simulink model "Milestone3"  (R2022a)
settings: Solver=FixedStepAuto  StartTime=0.0  StopTime=5000  RelTol=1e-3
undefined symbols (not defined in the file or in its folder): InputPWM, WheelSpeed
libraries: arduinolib x20, mobileRoboticsTrainingLib x2
settings Model: ExtModeTrigDuration=2  Creator=sarah  LastModifiedBy=sarah
settings OptimizationCC: EnhancedBackFolding=on  PassReuseOutputArgsAs=Individual arguments  ZeroExternalMemoryAtStartup=off  ZeroInternalMemoryAtStartup=off  MaxStackSize=64  OptimizeBlockOrder=speed  DifferentSizesBufferReuse=on  OptimizationCustomize=off  EfficientTunableParamExpr=on
settings DebuggingCC: ParameterTunabilityLossMsg=error
settings HardwareCC: ProdBitPerPointer=32  ProdBitPerSizeT=32  ProdBitPerPtrDiffT=32  ProdLargestAtomicInteger=Long  ProdLargestAtomicFloat=Double  ProdWordSize=32  ProdHWDeviceType=ARM Compatible->ARM Cortex  UseEmbeddedCoderFeatures=off  UseSimulinkCoderFeatures=off
settings SFSimCC: MATLABDynamicMemAlloc=off
settings RTWCC: SystemTargetFile=ert.tlc  HardwareBoard=Arduino Nano 33 IoT  TemplateMakefile=ert_default_tmf  Toolchain=Arduino ARM
settings CodeAppCC: ForceParamTrailComments=on  IgnoreCustomStorageClasses=off  OperatorAnnotations=on  SimulinkDataObjDesc=on  SFDataObjDesc=on  InsertBlockDesc=on
settings ERTTargetCC: SupportContinuousTime=on  SupportNonInlinedSFcns=on  SupportVariableSizeSignals=on  ExtModeTransport=3  ExtModeStaticAlloc=on  ExtModeStaticAllocSize=8192  ExtModeMexFile=ext_xcp  ExtModeIntrfLevel=Level2 - Open

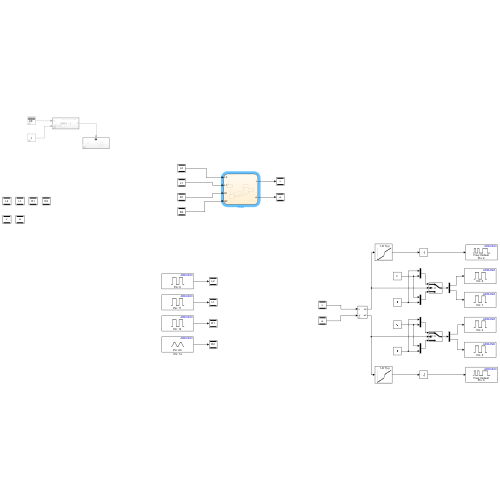
[thumbnail: Simulink's stored preview of the top-level diagram]
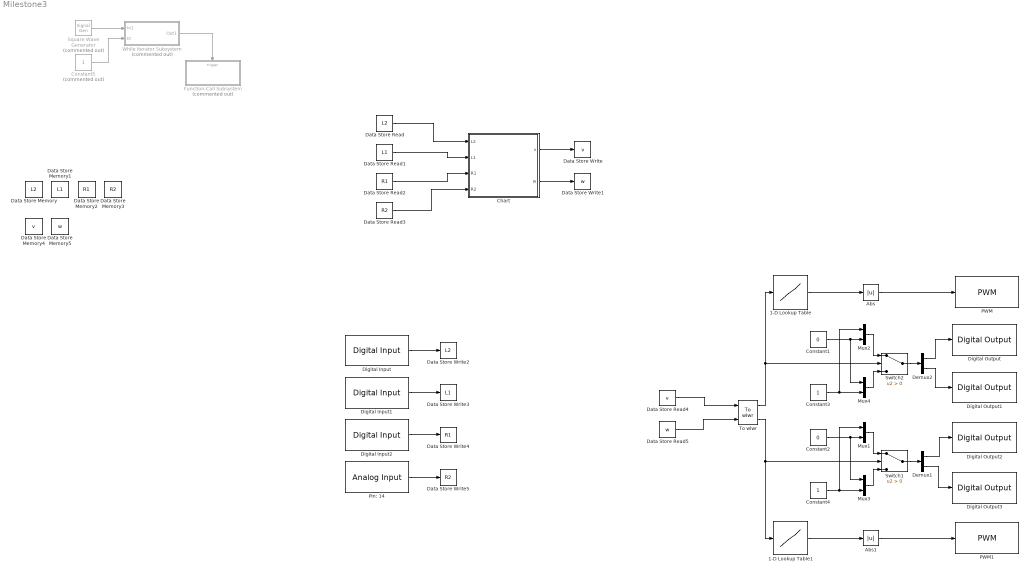
== system Milestone3 ==
  1-D Lookup Table : Lookup_n-D  NumberOfTableDimensions=1  BreakpointsForDimension1=WheelSpeed  Table=InputPWM  InternalRulePriority=Speed  RndMeth=Simplest
  1-D Lookup Table1 : Lookup_n-D  NumberOfTableDimensions=1  BreakpointsForDimension1=WheelSpeed  Table=InputPWM  InternalRulePriority=Speed  RndMeth=Simplest
  Abs : Abs  SaturateOnIntegerOverflow=off
  Abs1 : Abs  SaturateOnIntegerOverflow=off
  Chart : Stateflow chart  TreatAsAtomicUnit=on
  Constant1 : Constant  Value=0
  Constant2 : Constant  Value=0
  Constant3 : Constant
  Constant4 : Constant
  Constant5 : Constant  Commented=on
  Data Store Memory : DataStoreMemory  DataStoreName=L2  WriteAfterWriteMsg=warning  ShowAdditionalParam=off
  Data Store Memory1 : DataStoreMemory  DataStoreName=L1  WriteAfterWriteMsg=warning  ShowAdditionalParam=off
  Data Store Memory2 : DataStoreMemory  DataStoreName=R1  WriteAfterWriteMsg=warning  ShowAdditionalParam=off
  Data Store Memory3 : DataStoreMemory  DataStoreName=R2  WriteAfterWriteMsg=warning  ShowAdditionalParam=off
  Data Store Memory4 : DataStoreMemory  DataStoreName=v  WriteAfterWriteMsg=warning  ShowAdditionalParam=off
  Data Store Memory5 : DataStoreMemory  DataStoreName=w  WriteAfterWriteMsg=warning  ShowAdditionalParam=off
  Data Store Read : DataStoreRead  DataStoreName=L2  IndexOptions=Index vector (dialog)  Indices=1  OutputSizes=1
  Data Store Read1 : DataStoreRead  DataStoreName=L1  IndexOptions=Index vector (dialog)  Indices=1  OutputSizes=1
  Data Store Read2 : DataStoreRead  DataStoreName=R1  IndexOptions=Index vector (dialog)  Indices=1  OutputSizes=1
  Data Store Read3 : DataStoreRead  DataStoreName=R2  IndexOptions=Index vector (dialog)  Indices=1  OutputSizes=1
  Data Store Read4 : DataStoreRead  DataStoreName=v  IndexOptions=Index vector (dialog)  Indices=1  OutputSizes=1
  Data Store Read5 : DataStoreRead  DataStoreName=w  IndexOptions=Index vector (dialog)  Indices=1  OutputSizes=1
  Data Store Write : DataStoreWrite  DataStoreName=v  IndexOptions=Index vector (dialog)  Indices=1  OutputSizes=1
  Data Store Write1 : DataStoreWrite  DataStoreName=w  IndexOptions=Index vector (dialog)  Indices=1  OutputSizes=1
  Data Store Write2 : DataStoreWrite  DataStoreName=L2  IndexOptions=Index vector (dialog)  Indices=1  OutputSizes=1
  Data Store Write3 : DataStoreWrite  DataStoreName=L1  IndexOptions=Index vector (dialog)  Indices=1  OutputSizes=1
  Data Store Write4 : DataStoreWrite  DataStoreName=R1  IndexOptions=Index vector (dialog)  Indices=1  OutputSizes=1
  Data Store Write5 : DataStoreWrite  DataStoreName=R2  IndexOptions=Index vector (dialog)  Indices=1  OutputSizes=1
  Demux1 : Demux  Outputs=2
  Demux2 : Demux  Outputs=2
  Digital Input : arduinolib/Digital Input  pinNumber=8  mode=Default  Direction=input  SampleTime=-1  blockPlatform=arduino
  Digital Input1 : arduinolib/Digital Input  pinNumber=11  mode=Default  Direction=input  SampleTime=-1  blockPlatform=arduino
  Digital Input2 : arduinolib/Digital Input  pinNumber=12  mode=Default  Direction=input  SampleTime=-1  blockPlatform=arduino
  Digital Output : arduinolib/Digital Output  pinNumber=6  Direction=output  blockPlatform=arduino
  Digital Output1 : arduinolib/Digital Output  pinNumber=7  Direction=output  blockPlatform=arduino
  Digital Output2 : arduinolib/Digital Output  pinNumber=4  Direction=output  blockPlatform=arduino
  Digital Output3 : arduinolib/Digital Output  pinNumber=5  Direction=output  blockPlatform=arduino
  Function-Call Subsystem : Subsystem  Commented=on  TreatAsAtomicUnit=on
  Mux{1..4} (4 alike) : Mux  Inputs=2
  PWM : arduinolib/PWM  pinNumber=2  frequencyType=Default  desiredFrequency=490.2  achievableFrequency=490.2
  PWM1 : arduinolib/PWM  pinNumber=3  frequencyType=Default  desiredFrequency=490.2  achievableFrequency=490.2
  Pin: 14 : arduinolib/Analog Input  pinNumber=0  ReadResultsOnly=off  ConversionTriggerSource=Software  ExternalTriggerType=uint32( 0 )  OutputDataType=uint16  EnableConversionCompleteNotify=off  EnableOuputStatus=off  SampleTime=-1  blockPlatform=arduino
  Square Wave Generator : SignalGenerator  Commented=on  WaveForm=square  Units=rad/sec
  Switch1 : Switch  Criteria=u2 > Threshold  SaturateOnIntegerOverflow=off  InputSameDT=off
  Switch2 : Switch  Criteria=u2 > Threshold  SaturateOnIntegerOverflow=off  InputSameDT=off
  To wlwr : mobileRoboticsTrainingLib/To wlwr  axleLength=axleLength  wheelR=wheelR
  While Iterator Subsystem : Subsystem  Commented=on  TreatAsAtomicUnit=on
  wires:
  Square Wave Generator/1 -> While Iterator Subsystem/1(In1)
  Constant5/1 -> While Iterator Subsystem/2(IC)
  While Iterator Subsystem/1(Out1) -> Function-Call Subsystem/Trigger
  Chart/1(v) -> Data Store Write/1
  Chart/2(w) -> Data Store Write1/1
  Data Store Read/1 -> Chart/1(L2)
  Data Store Read1/1 -> Chart/2(L1)
  Data Store Read3/1 -> Chart/4(R2)
  Data Store Read2/1 -> Chart/3(R1)
  Pin: 14/1 -> Data Store Write5/1
  To wlwr/1 -> 1-D Lookup Table/1, Switch2/2
  Switch2/1 -> Demux2/1
  Constant1/1 -> Mux4/1, Mux2/2
  Abs1/1 -> PWM1/1
  Constant2/1 -> Mux3/1, Mux1/2
  Mux1/1 -> Switch1/1
  1-D Lookup Table1/1 -> Abs1/1
  Constant3/1 -> Mux2/1, Mux4/2
  Demux2/1 -> Digital Output/1
  Switch1/1 -> Demux1/1
  Abs/1 -> PWM/1
  Constant4/1 -> Mux1/1, Mux3/2
  Demux1/1 -> Digital Output2/1
  Demux1/2 -> Digital Output3/1
  To wlwr/2 -> Switch1/2, 1-D Lookup Table1/1
  Mux3/1 -> Switch1/3
  Mux4/1 -> Switch2/3
  Digital Input1/1 -> Data Store Write3/1
  Digital Input/1 -> Data Store Write2/1
  Mux2/1 -> Switch2/1
  Digital Input2/1 -> Data Store Write4/1
  Demux2/2 -> Digital Output1/1
  Data Store Read4/1 -> To wlwr/1
  1-D Lookup Table/1 -> Abs/1
  Data Store Read5/1 -> To wlwr/2

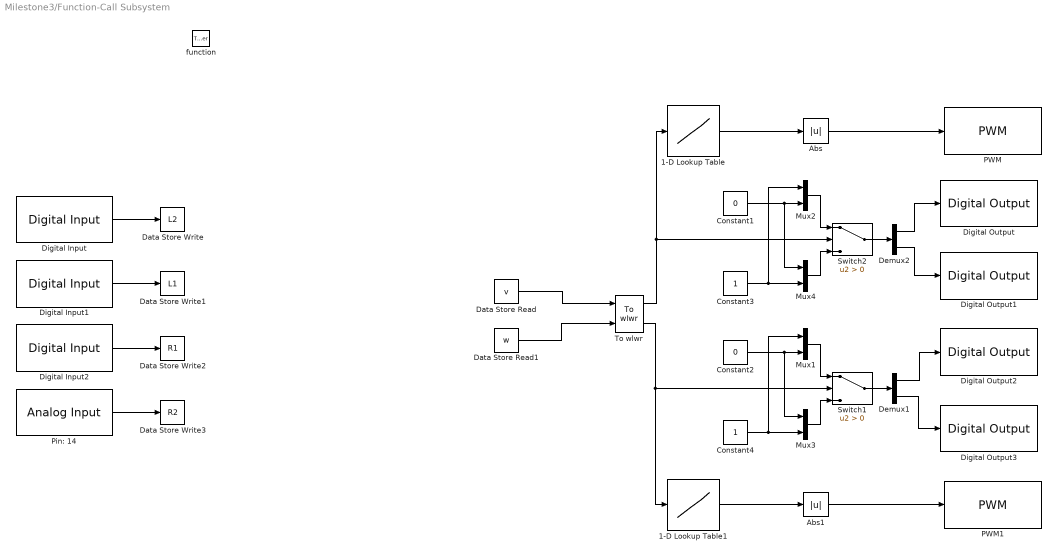
== system Milestone3/Function-Call Subsystem ==
  function : TriggerPort  TriggerType=either  VariantControl=(inherit)
  1-D Lookup Table : Lookup_n-D  NumberOfTableDimensions=1  BreakpointsForDimension1=WheelSpeed  Table=InputPWM  InternalRulePriority=Speed  RndMeth=Simplest
  1-D Lookup Table1 : Lookup_n-D  NumberOfTableDimensions=1  BreakpointsForDimension1=WheelSpeed  Table=InputPWM  InternalRulePriority=Speed  RndMeth=Simplest
  Abs : Abs  SaturateOnIntegerOverflow=off
  Abs1 : Abs  SaturateOnIntegerOverflow=off
  Constant1 : Constant  Value=0
  Constant2 : Constant  Value=0
  Constant3 : Constant
  Constant4 : Constant
  Data Store Read : DataStoreRead  DataStoreName=v  IndexOptions=Index vector (dialog)  Indices=1  OutputSizes=1
  Data Store Read1 : DataStoreRead  DataStoreName=w  IndexOptions=Index vector (dialog)  Indices=1  OutputSizes=1
  Data Store Write : DataStoreWrite  DataStoreName=L2  IndexOptions=Index vector (dialog)  Indices=1  OutputSizes=1
  Data Store Write1 : DataStoreWrite  DataStoreName=L1  IndexOptions=Index vector (dialog)  Indices=1  OutputSizes=1
  Data Store Write2 : DataStoreWrite  DataStoreName=R1  IndexOptions=Index vector (dialog)  Indices=1  OutputSizes=1
  Data Store Write3 : DataStoreWrite  DataStoreName=R2  IndexOptions=Index vector (dialog)  Indices=1  OutputSizes=1
  Demux1 : Demux  Outputs=2
  Demux2 : Demux  Outputs=2
  Digital Input : arduinolib/Digital Input  pinNumber=8  mode=Default  Direction=input  SampleTime=-1  blockPlatform=arduino
  Digital Input1 : arduinolib/Digital Input  pinNumber=11  mode=Default  Direction=input  SampleTime=-1  blockPlatform=arduino
  Digital Input2 : arduinolib/Digital Input  pinNumber=12  mode=Default  Direction=input  SampleTime=-1  blockPlatform=arduino
  Digital Output : arduinolib/Digital Output  pinNumber=6  Direction=output  blockPlatform=arduino
  Digital Output1 : arduinolib/Digital Output  pinNumber=7  Direction=output  blockPlatform=arduino
  Digital Output2 : arduinolib/Digital Output  pinNumber=4  Direction=output  blockPlatform=arduino
  Digital Output3 : arduinolib/Digital Output  pinNumber=5  Direction=output  blockPlatform=arduino
  Mux{1..4} (4 alike) : Mux  Inputs=2
  PWM : arduinolib/PWM  pinNumber=2  frequencyType=Default  desiredFrequency=490.2  achievableFrequency=490.2
  PWM1 : arduinolib/PWM  pinNumber=3  frequencyType=Default  desiredFrequency=490.2  achievableFrequency=490.2
  Pin: 14 : arduinolib/Analog Input  pinNumber=0  ReadResultsOnly=off  ConversionTriggerSource=Software  ExternalTriggerType=uint32( 0 )  OutputDataType=uint16  EnableConversionCompleteNotify=off  EnableOuputStatus=off  SampleTime=-1  blockPlatform=arduino
  Switch1 : Switch  Criteria=u2 > Threshold  SaturateOnIntegerOverflow=off  InputSameDT=off
  Switch2 : Switch  Criteria=u2 > Threshold  SaturateOnIntegerOverflow=off  InputSameDT=off
  To wlwr : mobileRoboticsTrainingLib/To wlwr  axleLength=axleLength  wheelR=wheelR
  wires:
  Digital Input/1 -> Data Store Write/1
  Pin: 14/1 -> Data Store Write3/1
  Digital Input2/1 -> Data Store Write2/1
  Digital Input1/1 -> Data Store Write1/1
  Constant3/1 -> Mux2/1, Mux4/2
  Constant2/1 -> Mux3/1, Mux1/2
  Constant1/1 -> Mux4/1, Mux2/2
  Abs1/1 -> PWM1/1
  Switch2/1 -> Demux2/1
  To wlwr/1 -> 1-D Lookup Table/1, Switch2/2
  Mux4/1 -> Switch2/3
  Mux3/1 -> Switch1/3
  Abs/1 -> PWM/1
  Demux1/1 -> Digital Output2/1
  Demux1/2 -> Digital Output3/1
  Demux2/1 -> Digital Output/1
  Switch1/1 -> Demux1/1
  Constant4/1 -> Mux1/1, Mux3/2
  1-D Lookup Table1/1 -> Abs1/1
  To wlwr/2 -> Switch1/2, 1-D Lookup Table1/1
  Mux1/1 -> Switch1/1
  Mux2/1 -> Switch2/1
  1-D Lookup Table/1 -> Abs/1
  Demux2/2 -> Digital Output1/1
  Data Store Read/1 -> To wlwr/1
  Data Store Read1/1 -> To wlwr/2

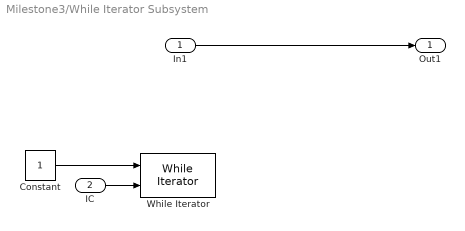
== system Milestone3/While Iterator Subsystem ==
  In1 : Inport
  IC : Inport  Port=2
  Constant : Constant
  While Iterator : WhileIterator
  Out1 : Outport
  wires:
  IC/1 -> While Iterator/2
  In1/1 -> Out1/1
  Constant/1 -> While Iterator/1

== stateflow chart Milestone3/Chart ==
  state Begin
    entry:
    v = 0;
  state AdjustRight
    entry:
    w =- 0.6;
  state AdjustLeft
    entry:
    w = 0.7;
  state Start
    entry:
    v = 0.06;
    w = 0.05;
  (default) -> Begin : %start
  Start -> AdjustRight [order 2] : [L2&&L1&&~R1&&R2]
  AdjustRight -> Start : [(L1&&R1)==0]
  Begin -> Start : [(L1&&R1)==0]
  Start -> AdjustLeft [order 1] : [L2&&~L1&&R1&&R2]
  AdjustLeft -> Start : [(L1&&R1)==0]
  data: L2 input; L1 input; R1 input; R2 input; v output; w output
